simulink model "MMotorMax"  (R2024b)
settings: configuration reference "STM32H7_Config" (kept outside this file)
undefined symbols (not defined in the file): MMotorMaxAllowed, MNominal, PMotorMaxAllowed
settings Model: DataDictionary=Master_Dictionary.sldd  EnableAccessToBaseWorkspace=off  Creator=torni  LastModifiedBy=Will
settings ConfigSetRef: SourceName=STM32H7_Config

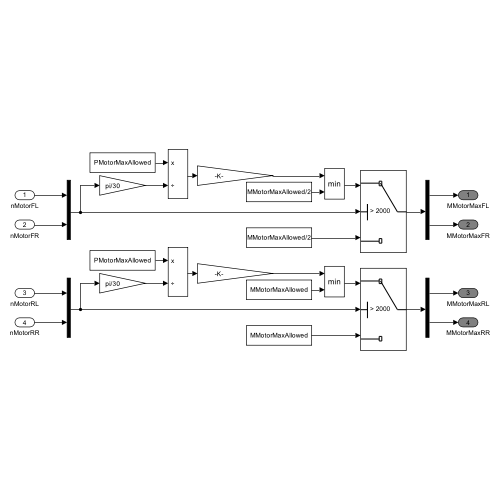
[thumbnail: Simulink's stored preview of the top-level diagram]
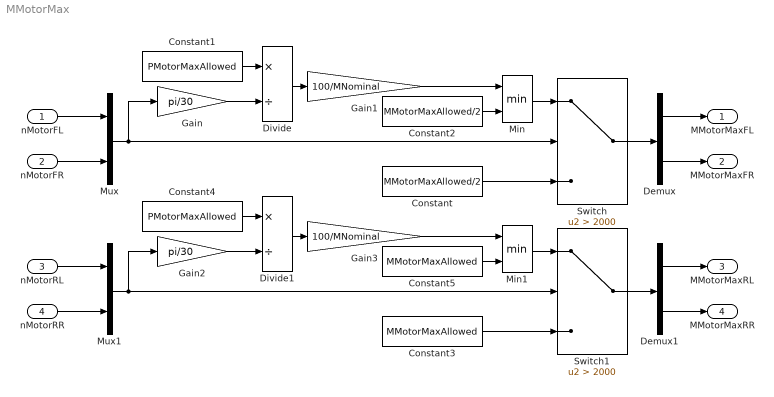
== system MMotorMax ==
  nMotorFL : Inport  OutDataTypeStr=double
  nMotorFR : Inport  Port=2  OutDataTypeStr=double
  nMotorRL : Inport  Port=3  OutDataTypeStr=double
  nMotorRR : Inport  Port=4  OutDataTypeStr=double
  Constant : Constant  Value=MMotorMaxAllowed/2
  Constant1 : Constant  Value=PMotorMaxAllowed
  Constant2 : Constant  Value=MMotorMaxAllowed/2
  Constant3 : Constant  Value=MMotorMaxAllowed
  Constant4 : Constant  Value=PMotorMaxAllowed
  Constant5 : Constant  Value=MMotorMaxAllowed
  Demux : Demux  Outputs=2
  Demux1 : Demux  Outputs=2
  Divide : Product  Inputs=*/  RndMeth=Zero  SaturateOnIntegerOverflow=on
  Divide1 : Product  Inputs=*/  RndMeth=Zero  SaturateOnIntegerOverflow=on
  Gain : Gain  Gain=pi/30
  Gain1 : Gain  Gain=100/MNominal
  Gain2 : Gain  Gain=pi/30
  Gain3 : Gain  Gain=100/MNominal
  Min : MinMax  Inputs=2
  Min1 : MinMax  Inputs=2
  Mux : Mux  Inputs=2
  Mux1 : Mux  Inputs=2
  Switch : Switch  Criteria=u2 > Threshold  Threshold=2000  SaturateOnIntegerOverflow=off  InputSameDT=off
  Switch1 : Switch  Criteria=u2 > Threshold  Threshold=2000  SaturateOnIntegerOverflow=off  InputSameDT=off
  MMotorMaxFL : Outport  OutDataTypeStr=double  VectorParamsAs1DForOutWhenUnconnected=off
  MMotorMaxFR : Outport  Port=2  OutDataTypeStr=double  VectorParamsAs1DForOutWhenUnconnected=off
  MMotorMaxRL : Outport  Port=3  OutDataTypeStr=double  VectorParamsAs1DForOutWhenUnconnected=off
  MMotorMaxRR : Outport  Port=4  OutDataTypeStr=double  VectorParamsAs1DForOutWhenUnconnected=off
  wires:
  nMotorFL/1 -> Mux/1
  nMotorFR/1 -> Mux/2
  Switch/1 -> Demux/1
  Constant/1 -> Switch/3
  Mux/1 -> Gain/1, Switch/2
  Gain/1 -> Divide/2
  Constant1/1 -> Divide/1
  Divide/1 -> Gain1/1
  Min/1 -> Switch/1
  Constant2/1 -> Min/2
  Gain1/1 -> Min/1
  Demux/2 -> MMotorMaxFR/1
  Demux/1 -> MMotorMaxFL/1
  Demux1/1 -> MMotorMaxRL/1
  Demux1/2 -> MMotorMaxRR/1
  Gain3/1 -> Min1/1
  Constant5/1 -> Min1/2
  Min1/1 -> Switch1/1
  Divide1/1 -> Gain3/1
  Constant4/1 -> Divide1/1
  Gain2/1 -> Divide1/2
  Mux1/1 -> Switch1/2, Gain2/1
  Constant3/1 -> Switch1/3
  Switch1/1 -> Demux1/1
  nMotorRR/1 -> Mux1/2
  nMotorRL/1 -> Mux1/1
